simulink model "OldController"  (R2021b)
settings: Solver=VariableStepAuto  StartTime=0.0  StopTime=10.0  RelTol=1e-3
undefined symbols (not defined in the file or in its folder): K
settings Model: Creator=17165  LastModifiedBy=17165

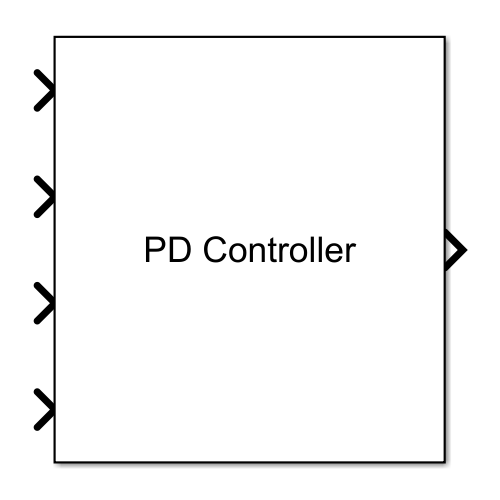
[thumbnail: Simulink's stored preview of the top-level diagram]
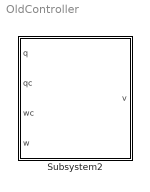
== system OldController ==
  Subsystem2 : Subsystem
      mask Display: disp('PD Controller')

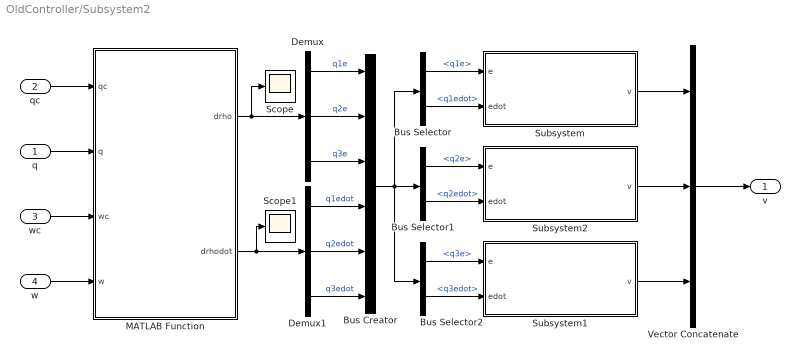
== system OldController/Subsystem2 ==
  q : Inport
  qc : Inport  Port=2
  wc : Inport  Port=3
  w : Inport  Port=4
  Bus Creator : BusCreator  Inputs=6
  Bus Selector : BusSelector  OutputSignals=q1e,q1edot
  Bus Selector1 : BusSelector  OutputSignals=q2e,q2edot
  Bus Selector2 : BusSelector  OutputSignals=q3e,q3edot
  Demux : Demux  Outputs=3
  Demux1 : Demux  Outputs=3
  MATLAB Function : MATLAB Function  TreatAsAtomicUnit=on
  Scope : Scope
  Scope1 : Scope
  Subsystem : Subsystem  mask{Kp=K(1), Kd=K(2)}
      mask Display: disp('PD-Compensator')
  Subsystem1 : Subsystem  mask{Kp=K(1), Kd=K(2)}
      mask Display: disp('PD-Compensator')
  Subsystem2 : Subsystem  mask{Kp=K(1), Kd=K(2)}
      mask Display: disp('PD-Compensator')
  Vector Concatenate : Concatenate  NumInputs=3
  v : Outport
  wires:
  Vector Concatenate/1 -> v/1
  Subsystem/1(v) -> Vector Concatenate/1
  Subsystem2/1(v) -> Vector Concatenate/2
  Subsystem1/1(v) -> Vector Concatenate/3
  MATLAB Function/1(drho) -> Scope/1, Demux/1
  MATLAB Function/2(drhodot) -> Scope1/1, Demux1/1
  Demux/1 -> Bus Creator/1  "q1e"
  Demux/2 -> Bus Creator/2  "q2e"
  Demux/3 -> Bus Creator/3  "q3e"
  Demux1/1 -> Bus Creator/4  "q1edot"
  Demux1/2 -> Bus Creator/5  "q2edot"
  Demux1/3 -> Bus Creator/6  "q3edot"
  Bus Selector/1 -> Subsystem/1(e)  "<q1e>"
  Bus Selector/2 -> Subsystem/2(edot)  "<q1edot>"
  Bus Selector2/2 -> Subsystem1/2(edot)  "<q3edot>"
  Bus Selector2/1 -> Subsystem1/1(e)  "<q3e>"
  Bus Selector1/1 -> Subsystem2/1(e)  "<q2e>"
  Bus Selector1/2 -> Subsystem2/2(edot)  "<q2edot>"
  Bus Creator/1 -> Bus Selector2/1, Bus Selector/1, Bus Selector1/1
  q/1 -> MATLAB Function/2(q)
  qc/1 -> MATLAB Function/1(qc)
  wc/1 -> MATLAB Function/3(wc)
  w/1 -> MATLAB Function/4(w)

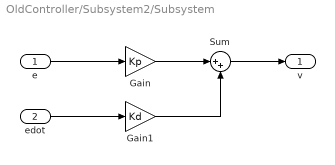
== system OldController/Subsystem2/Subsystem ==
  e : Inport
  edot : Inport  Port=2
  Gain : Gain  Gain=Kp
  Gain1 : Gain  Gain=Kd
  Sum : Sum  Inputs=|++
  v : Outport
  wires:
  e/1 -> Gain/1
  Gain/1 -> Sum/1
  edot/1 -> Gain1/1
  Gain1/1 -> Sum/2
  Sum/1 -> v/1

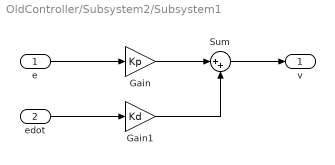
== system OldController/Subsystem2/Subsystem1 ==
  e : Inport
  edot : Inport  Port=2
  Gain : Gain  Gain=Kp
  Gain1 : Gain  Gain=Kd
  Sum : Sum  Inputs=|++
  v : Outport
  wires:
  e/1 -> Gain/1
  Gain/1 -> Sum/1
  edot/1 -> Gain1/1
  Gain1/1 -> Sum/2
  Sum/1 -> v/1

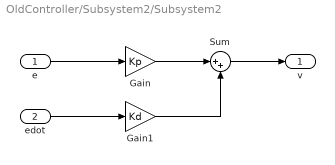
== system OldController/Subsystem2/Subsystem2 ==
  e : Inport
  edot : Inport  Port=2
  Gain : Gain  Gain=Kp
  Gain1 : Gain  Gain=Kd
  Sum : Sum  Inputs=|++
  v : Outport
  wires:
  e/1 -> Gain/1
  Gain/1 -> Sum/1
  edot/1 -> Gain1/1
  Gain1/1 -> Sum/2
  Sum/1 -> v/1

== matlab function OldController/Subsystem2/MATLAB Function ==
  data: qc input; drho output; q input; drhodot output; wc input; w input
function [drho,drhodot] = QuaternionErrorDynamics(qc,q,wc,w)
drho        = zeros(3,1);
drhodot     = zeros(3,1);
dq          = QuaternionError(qc,q);

% Quaternion Error Rate, Crassidis & Markley 8.66a
drho        = dq(1:3,1);
dw          = w - wc;
drhodot     = -cross(w,drho) + (1/2)*(dq(4,1)*dw - cross(dw,drho));
end
